simulink model "BrowarModel"  (R2024a)
settings: Solver=ode5  StartTime=0.0  StopTime=inf  FixedStep=0.1  RelTol=1e-3
undefined symbols (not defined in the file or in its folder): localhost, Matrikon, OI
libraries: opclib x24
(part 2 of 9)

== system BrowarModel/Kadz fermentacyjna/ET705 ==
  note: Przetwornik pomiarowy
  In : Inport
  F_gain : Gain  Gain=0
  F_offset : Constant  Value=0
  GUIMon : Gain
  Kompensacja : Constant  Value=Kompensacja
  Product : Product  RndMeth=Zero
  Saturation : Saturate  UpperLimit=100  LowerLimit=0
  Skalowanie (0-100%) : Gain  Gain=100/SrcZakres
  Sum{,1..3} (4 alike) : Sum  Inputs=|++
  Transfer Fcn : TransferFcn  Denominator=[0.3 1]
  Zaklocenia pomiarowe : Subsystem
  Zakres : Constant  Value=Zakres/100
  Out : Outport
  wires:
  Saturation/1 -> Product/1
  GUIMon/1 -> Out/1
  In/1 -> Skalowanie (0-100%)/1
  Sum2/1 -> Sum3/1
  Sum3/1 -> Transfer Fcn/1
  Sum1/1 -> Sum2/1, F_gain/1
  Zaklocenia pomiarowe/1(Out) -> Sum1/2
  Skalowanie (0-100%)/1 -> Sum1/1
  Sum/1 -> GUIMon/1
  Kompensacja/1 -> Sum/2
  Zakres/1 -> Product/2
  Product/1 -> Sum/1
  F_gain/1 -> Sum2/2
  F_offset/1 -> Sum3/2
  Transfer Fcn/1 -> Saturation/1

== system BrowarModel/Kadz fermentacyjna/FV705 ==
  note: Sterowanie
  GUIMon : Gain
  Lokalne : Constant
  Wybor : Switch  Threshold=0.5  SaturateOnIntegerOverflow=off  InputSameDT=off
  Out : Outport
  wires:
  GUIMon/1 -> Out/1
  Wybor/1 -> GUIMon/1
  [TrybSter] -> Wybor/2
  [FV705] -> Wybor/1
  Lokalne/1 -> Wybor/3

== system BrowarModel/Kadz fermentacyjna/FV705SP ==
  note: Sterowanie
  GUIMon : Gain
  Lokalne : Constant  Value=100
  Wybor : Switch  Threshold=0.5  SaturateOnIntegerOverflow=off  InputSameDT=off
  Out : Outport
  wires:
  Lokalne/1 -> Wybor/3
  [FV705SP] -> Wybor/1
  [TrybSter] -> Wybor/2
  Wybor/1 -> GUIMon/1
  GUIMon/1 -> Out/1

== system BrowarModel/Kadz fermentacyjna/FV706 ==
  note: Sterowanie
  GUIMon : Gain
  Lokalne : Constant
  Wybor : Switch  Threshold=0.5  SaturateOnIntegerOverflow=off  InputSameDT=off
  Out : Outport
  wires:
  GUIMon/1 -> Out/1
  Wybor/1 -> GUIMon/1
  [TrybSter] -> Wybor/2
  [FV706] -> Wybor/1
  Lokalne/1 -> Wybor/3

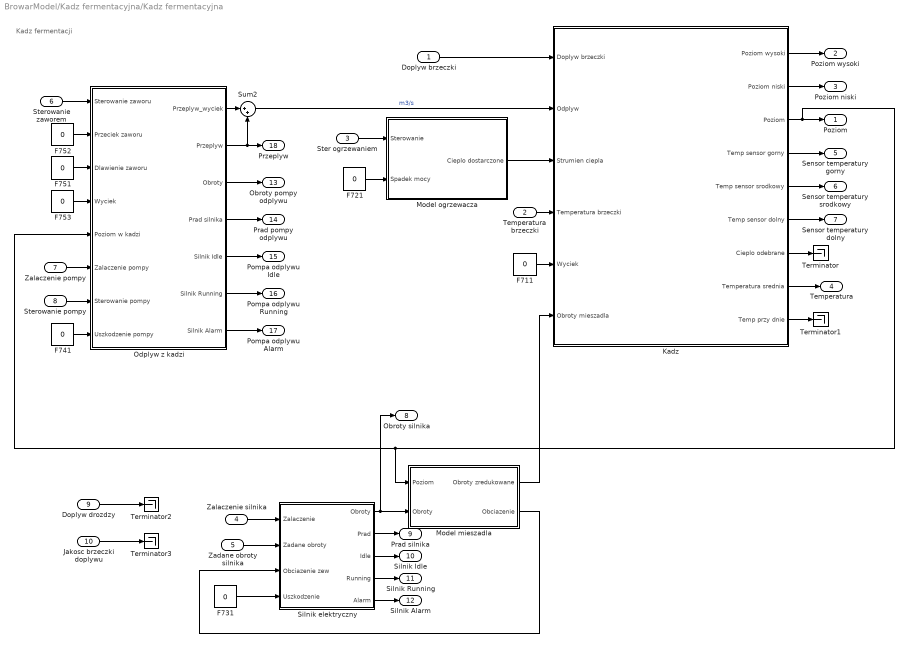
== system BrowarModel/Kadz fermentacyjna/Kadz fermentacyjna ==
  note: Kadz fermentacji
  Doplyw brzeczki : Inport
  Temperatura brzeczki : Inport  Port=2
  Ster ogrzewaniem : Inport  Port=3
  Zalaczenie silnika : Inport  Port=4
  "Zadane obroty silnika " : Inport  Port=5
  Sterowanie zaworem : Inport  Port=6
  Zalaczenie pompy : Inport  Port=7
  Sterowanie pompy : Inport  Port=8
  Doplyw drozdzy : Inport  Port=9
  Jakosc brzeczki doplywu : Inport  Port=10
  F{711,721,731,741,751..753} (7 alike) : Constant  Value=0
  Kadz : Subsystem
  Model mieszadla : Subsystem
  Model ogrzewacza : Subsystem
  Odplyw z kadzi : Subsystem
  Silnik elektryczny : Subsystem
  Sum2 : Sum  Inputs=|++
  Terminator{,1..3} (4 alike) : Terminator
  Poziom : Outport
  Poziom wysoki : Outport  Port=2
  Poziom niski : Outport  Port=3
  Temperatura : Outport  Port=4
  Sensor temperatury gorny : Outport  Port=5
  Sensor temperatury srodkowy : Outport  Port=6
  Sensor temperatury dolny : Outport  Port=7
  Obroty silnika : Outport  Port=8
  Prad silnika : Outport  Port=9
  Silnik Idle : Outport  Port=10
  Silnik Running : Outport  Port=11
  Silnik Alarm : Outport  Port=12
  Obroty pompy odplywu : Outport  Port=13
  Prad pompy odplywu : Outport  Port=14
  Pompa odplywu Idle : Outport  Port=15
  Pompa odplywu Running : Outport  Port=16
  Pompa odplywu Alarm : Outport  Port=17
  Przeplyw : Outport  Port=18
  wires:
  Model ogrzewacza/1(Cieplo dostarczone) -> Kadz/3(Strumien ciepla)
  Kadz/6(Temp sensor dolny) -> Sensor temperatury dolny/1
  Kadz/5(Temp sensor srodkowy) -> Sensor temperatury srodkowy/1
  Kadz/4(Temp sensor gorny) -> Sensor temperatury gorny/1
  Kadz/2(Poziom niski) -> Poziom niski/1
  Kadz/1(Poziom wysoki) -> Poziom wysoki/1
  Doplyw brzeczki/1 -> Kadz/1(Doplyw brzeczki)
  Temperatura brzeczki/1 -> Kadz/4(Temperatura brzeczki)
  Model mieszadla/1(Obroty zredukowane) -> Kadz/6(Obroty mieszadla)
  Kadz/3(Poziom) -> Poziom/1, Model mieszadla/1(Poziom), Odplyw z kadzi/5(Poziom w kadzi)
  Sum2/1 -> Kadz/2(Odplyw)  "m3/s"
  Kadz/8(Temperatura srednia) -> Temperatura/1
  F711/1 -> Kadz/5(Wyciek)
  Kadz/7(Cieplo odebrane) -> Terminator/1
  Silnik elektryczny/1(Obroty) -> Obroty silnika/1, Model mieszadla/2(Obroty)
  Ster ogrzewaniem/1 -> Model ogrzewacza/1(Sterowanie)
  F721/1 -> Model ogrzewacza/2(Spadek mocy)
  Kadz/9(Temp przy dnie) -> Terminator1/1
  Silnik elektryczny/3(Idle) -> Silnik Idle/1
  Silnik elektryczny/4(Running) -> Silnik Running/1
  Silnik elektryczny/5(Alarm) -> Silnik Alarm/1
  Silnik elektryczny/2(Prad) -> Prad silnika/1
  F731/1 -> Silnik elektryczny/4(Uszkodzenie)
  "Zadane obroty silnika "/1 -> Silnik elektryczny/2(Zadane obroty)
  Zalaczenie silnika/1 -> Silnik elektryczny/1(Zalaczenie)
  F752/1 -> Odplyw z kadzi/2(Przeciek zaworu)
  F751/1 -> Odplyw z kadzi/3(Dlawienie zaworu)
  F741/1 -> Odplyw z kadzi/8(Uszkodzenie pompy)
  Sterowanie zaworem/1 -> Odplyw z kadzi/1(Sterowanie zaworu)
  Zalaczenie pompy/1 -> Odplyw z kadzi/6(Zalaczenie pompy)
  Sterowanie pompy/1 -> Odplyw z kadzi/7(Sterowanie pompy)
  F753/1 -> Odplyw z kadzi/4(Wyciek)
  Odplyw z kadzi/4(Prad silnika) -> Prad pompy odplywu/1
  Odplyw z kadzi/5(Silnik Idle) -> Pompa odplywu Idle/1
  Odplyw z kadzi/6(Silnik Running) -> Pompa odplywu Running/1
  Odplyw z kadzi/7(Silnik Alarm) -> Pompa odplywu Alarm/1
  Odplyw z kadzi/3(Obroty) -> Obroty pompy odplywu/1
  Odplyw z kadzi/2(Przeplyw) -> Sum2/2, Przeplyw/1
  Odplyw z kadzi/1(Przeplyw_wyciek) -> Sum2/1
  Model mieszadla/2(Obciazenie) -> Silnik elektryczny/3(Obciazenie zew)
  Doplyw drozdzy/1 -> Terminator2/1
  Jakosc brzeczki doplywu/1 -> Terminator3/1

== system BrowarModel/Kadz fermentacyjna/LT701 ==
  note: Przetwornik pomiarowy
  In : Inport
  F_gain : Gain  Gain=0
  F_offset : Constant  Value=0
  GUIMon : Gain
  Kompensacja : Constant  Value=Kompensacja
  Product : Product  RndMeth=Zero
  Saturation : Saturate  UpperLimit=100  LowerLimit=0
  Skalowanie (0-100%) : Gain  Gain=100/SrcZakres
  Sum{,1..3} (4 alike) : Sum  Inputs=|++
  Transfer Fcn : TransferFcn  Denominator=[0.3 1]
  Zaklocenia pomiarowe : Subsystem
  Zakres : Constant  Value=Zakres/100
  Out : Outport
  wires:
  Saturation/1 -> Product/1
  GUIMon/1 -> Out/1
  In/1 -> Skalowanie (0-100%)/1
  Sum2/1 -> Sum3/1
  Sum3/1 -> Transfer Fcn/1
  Sum1/1 -> Sum2/1, F_gain/1
  Zaklocenia pomiarowe/1(Out) -> Sum1/2
  Skalowanie (0-100%)/1 -> Sum1/1
  Sum/1 -> GUIMon/1
  Kompensacja/1 -> Sum/2
  Zakres/1 -> Product/2
  Product/1 -> Sum/1
  F_gain/1 -> Sum2/2
  F_offset/1 -> Sum3/2
  Transfer Fcn/1 -> Saturation/1

== system BrowarModel/Kadz fermentacyjna/LT701H ==
  note: Przetwornik pomiarowy
  In : Inport
  FT : Constant  Value=0
  FT_value : Constant  Value=0
  GUIMon : Gain
  Switch : Switch  Threshold=0.5  SaturateOnIntegerOverflow=off  InputSameDT=off
  Out : Outport
  wires:
  In/1 -> Switch/3
  GUIMon/1 -> Out/1
  FT/1 -> Switch/2
  Switch/1 -> GUIMon/1
  FT_value/1 -> Switch/1

== system BrowarModel/Kadz fermentacyjna/LT701L ==
  note: Przetwornik pomiarowy
  In : Inport
  FT : Constant  Value=0
  FT_value : Constant  Value=0
  GUIMon : Gain
  Switch : Switch  Threshold=0.5  SaturateOnIntegerOverflow=off  InputSameDT=off
  Out : Outport
  wires:
  FT_value/1 -> Switch/1
  Switch/1 -> GUIMon/1
  FT/1 -> Switch/2
  GUIMon/1 -> Out/1
  In/1 -> Switch/3

== system BrowarModel/Kadz fermentacyjna/ST704 ==
  note: Przetwornik pomiarowy
  In : Inport
  F_gain : Gain  Gain=0
  F_offset : Constant  Value=0
  GUIMon : Gain
  Kompensacja : Constant  Value=Kompensacja
  Product : Product  RndMeth=Zero
  Saturation : Saturate  UpperLimit=100  LowerLimit=0
  Skalowanie (0-100%) : Gain  Gain=100/SrcZakres
  Sum{,1..3} (4 alike) : Sum  Inputs=|++
  Transfer Fcn : TransferFcn  Denominator=[0.3 1]
  Zaklocenia pomiarowe : Subsystem
  Zakres : Constant  Value=Zakres/100
  Out : Outport
  wires:
  Saturation/1 -> Product/1
  GUIMon/1 -> Out/1
  In/1 -> Skalowanie (0-100%)/1
  Sum2/1 -> Sum3/1
  Sum3/1 -> Transfer Fcn/1
  Sum1/1 -> Sum2/1, F_gain/1
  Zaklocenia pomiarowe/1(Out) -> Sum1/2
  Skalowanie (0-100%)/1 -> Sum1/1
  Sum/1 -> GUIMon/1
  Kompensacja/1 -> Sum/2
  Zakres/1 -> Product/2
  Product/1 -> Sum/1
  F_gain/1 -> Sum2/2
  F_offset/1 -> Sum3/2
  Transfer Fcn/1 -> Saturation/1

== system BrowarModel/Kadz fermentacyjna/ST705 ==
  note: Przetwornik pomiarowy
  In : Inport
  F_gain : Gain  Gain=0
  F_offset : Constant  Value=0
  GUIMon : Gain
  Kompensacja : Constant  Value=Kompensacja
  Product : Product  RndMeth=Zero
  Saturation : Saturate  UpperLimit=100  LowerLimit=0
  Skalowanie (0-100%) : Gain  Gain=100/SrcZakres
  Sum{,1..3} (4 alike) : Sum  Inputs=|++
  Transfer Fcn : TransferFcn  Denominator=[0.3 1]
  Zaklocenia pomiarowe : Subsystem
  Zakres : Constant  Value=Zakres/100
  Out : Outport
  wires:
  Transfer Fcn/1 -> Saturation/1
  F_offset/1 -> Sum3/2
  F_gain/1 -> Sum2/2
  Product/1 -> Sum/1
  Zakres/1 -> Product/2
  Kompensacja/1 -> Sum/2
  Sum/1 -> GUIMon/1
  Skalowanie (0-100%)/1 -> Sum1/1
  Zaklocenia pomiarowe/1(Out) -> Sum1/2
  Sum1/1 -> F_gain/1, Sum2/1
  Sum3/1 -> Transfer Fcn/1
  Sum2/1 -> Sum3/1
  In/1 -> Skalowanie (0-100%)/1
  GUIMon/1 -> Out/1
  Saturation/1 -> Product/1

== system BrowarModel/Kadz fermentacyjna/TT702H ==
  note: Przetwornik pomiarowy
  In : Inport
  F_gain : Gain  Gain=0
  F_offset : Constant  Value=0
  GUIMon : Gain
  Kompensacja : Constant  Value=Kompensacja
  Product : Product  RndMeth=Zero
  Saturation : Saturate  UpperLimit=100  LowerLimit=0
  Skalowanie (0-100%) : Gain  Gain=100/SrcZakres
  Sum{,1..3} (4 alike) : Sum  Inputs=|++
  Transfer Fcn : TransferFcn  Denominator=[0.3 1]
  Zaklocenia pomiarowe : Subsystem
  Zakres : Constant  Value=Zakres/100
  Out : Outport
  wires:
  Transfer Fcn/1 -> Saturation/1
  F_offset/1 -> Sum3/2
  F_gain/1 -> Sum2/2
  Product/1 -> Sum/1
  Zakres/1 -> Product/2
  Kompensacja/1 -> Sum/2
  Sum/1 -> GUIMon/1
  Skalowanie (0-100%)/1 -> Sum1/1
  Zaklocenia pomiarowe/1(Out) -> Sum1/2
  Sum1/1 -> F_gain/1, Sum2/1
  Sum3/1 -> Transfer Fcn/1
  Sum2/1 -> Sum3/1
  In/1 -> Skalowanie (0-100%)/1
  GUIMon/1 -> Out/1
  Saturation/1 -> Product/1

== system BrowarModel/Kadz fermentacyjna/TT702L ==
  note: Przetwornik pomiarowy
  In : Inport
  F_gain : Gain  Gain=0
  F_offset : Constant  Value=0
  GUIMon : Gain
  Kompensacja : Constant  Value=Kompensacja
  Product : Product  RndMeth=Zero
  Saturation : Saturate  UpperLimit=100  LowerLimit=0
  Skalowanie (0-100%) : Gain  Gain=100/SrcZakres
  Sum{,1..3} (4 alike) : Sum  Inputs=|++
  Transfer Fcn : TransferFcn  Denominator=[0.3 1]
  Zaklocenia pomiarowe : Subsystem
  Zakres : Constant  Value=Zakres/100
  Out : Outport
  wires:
  Transfer Fcn/1 -> Saturation/1
  F_offset/1 -> Sum3/2
  F_gain/1 -> Sum2/2
  Product/1 -> Sum/1
  Zakres/1 -> Product/2
  Kompensacja/1 -> Sum/2
  Sum/1 -> GUIMon/1
  Skalowanie (0-100%)/1 -> Sum1/1
  Zaklocenia pomiarowe/1(Out) -> Sum1/2
  Sum1/1 -> F_gain/1, Sum2/1
  Sum3/1 -> Transfer Fcn/1
  Sum2/1 -> Sum3/1
  In/1 -> Skalowanie (0-100%)/1
  GUIMon/1 -> Out/1
  Saturation/1 -> Product/1

== system BrowarModel/Kadz fermentacyjna/TT702M ==
  note: Przetwornik pomiarowy
  In : Inport
  F_gain : Gain  Gain=0
  F_offset : Constant  Value=0
  GUIMon : Gain
  Kompensacja : Constant  Value=Kompensacja
  Product : Product  RndMeth=Zero
  Saturation : Saturate  UpperLimit=100  LowerLimit=0
  Skalowanie (0-100%) : Gain  Gain=100/SrcZakres
  Sum{,1..3} (4 alike) : Sum  Inputs=|++
  Transfer Fcn : TransferFcn  Denominator=[0.3 1]
  Zaklocenia pomiarowe : Subsystem
  Zakres : Constant  Value=Zakres/100
  Out : Outport
  wires:
  Saturation/1 -> Product/1
  GUIMon/1 -> Out/1
  In/1 -> Skalowanie (0-100%)/1
  Sum2/1 -> Sum3/1
  Sum3/1 -> Transfer Fcn/1
  Sum1/1 -> Sum2/1, F_gain/1
  Zaklocenia pomiarowe/1(Out) -> Sum1/2
  Skalowanie (0-100%)/1 -> Sum1/1
  Sum/1 -> GUIMon/1
  Kompensacja/1 -> Sum/2
  Zakres/1 -> Product/2
  Product/1 -> Sum/1
  F_gain/1 -> Sum2/2
  F_offset/1 -> Sum3/2
  Transfer Fcn/1 -> Saturation/1

== system BrowarModel/Kadz fermentacyjna/TV702 ==
  note: Sterowanie
  GUIMon : Gain
  Lokalne : Constant  Value=0
  Wybor : Switch  Threshold=0.5  SaturateOnIntegerOverflow=off  InputSameDT=off
  Out : Outport
  wires:
  GUIMon/1 -> Out/1
  Wybor/1 -> GUIMon/1
  [TrybSter] -> Wybor/2
  [TV702] -> Wybor/1
  Lokalne/1 -> Wybor/3

== system BrowarModel/Kadz fermentacyjna/XV704 ==
  note: Sterowanie
  GUIMon : Gain
  Lokalne : Constant
  Wybor : Switch  Threshold=0.5  SaturateOnIntegerOverflow=off  InputSameDT=off
  Out : Outport
  wires:
  Lokalne/1 -> Wybor/3
  [XV704] -> Wybor/1
  [TrybSter] -> Wybor/2
  Wybor/1 -> GUIMon/1
  GUIMon/1 -> Out/1

== system BrowarModel/Kadz fermentacyjna/XV704SP ==
  note: Sterowanie
  GUIMon : Gain
  Lokalne : Constant  Value=100
  Wybor : Switch  Threshold=0.5  SaturateOnIntegerOverflow=off  InputSameDT=off
  Out : Outport
  wires:
  GUIMon/1 -> Out/1
  Wybor/1 -> GUIMon/1
  [TrybSter] -> Wybor/2
  [XV704SP] -> Wybor/1
  Lokalne/1 -> Wybor/3

== system BrowarModel/Kadz filtracji/ET302 ==
  note: Przetwornik pomiarowy
  In : Inport
  F_gain : Gain  Gain=0
  F_offset : Constant  Value=0
  GUIMon : Gain
  Kompensacja : Constant  Value=Kompensacja
  Product : Product  RndMeth=Zero
  Saturation : Saturate  UpperLimit=100  LowerLimit=0
  Skalowanie (0-100%) : Gain  Gain=100/SrcZakres
  Sum{,1..3} (4 alike) : Sum  Inputs=|++
  Transfer Fcn : TransferFcn  Denominator=[0.3 1]
  Zaklocenia pomiarowe : Subsystem
  Zakres : Constant  Value=Zakres/100
  Out : Outport
  wires:
  Transfer Fcn/1 -> Saturation/1
  F_offset/1 -> Sum3/2
  F_gain/1 -> Sum2/2
  Product/1 -> Sum/1
  Zakres/1 -> Product/2
  Kompensacja/1 -> Sum/2
  Sum/1 -> GUIMon/1
  Skalowanie (0-100%)/1 -> Sum1/1
  Zaklocenia pomiarowe/1(Out) -> Sum1/2
  Sum1/1 -> F_gain/1, Sum2/1
  Sum3/1 -> Transfer Fcn/1
  Sum2/1 -> Sum3/1
  In/1 -> Skalowanie (0-100%)/1
  GUIMon/1 -> Out/1
  Saturation/1 -> Product/1

== system BrowarModel/Kadz filtracji/ET304 ==
  note: Przetwornik pomiarowy
  In : Inport
  F_gain : Gain  Gain=0
  F_offset : Constant  Value=0
  GUIMon : Gain
  Kompensacja : Constant  Value=Kompensacja
  Product : Product  RndMeth=Zero
  Saturation : Saturate  UpperLimit=100  LowerLimit=0
  Skalowanie (0-100%) : Gain  Gain=100/SrcZakres
  Sum{,1..3} (4 alike) : Sum  Inputs=|++
  Transfer Fcn : TransferFcn  Denominator=[0.3 1]
  Zaklocenia pomiarowe : Subsystem
  Zakres : Constant  Value=Zakres/100
  Out : Outport
  wires:
  Saturation/1 -> Product/1
  GUIMon/1 -> Out/1
  In/1 -> Skalowanie (0-100%)/1
  Sum2/1 -> Sum3/1
  Sum3/1 -> Transfer Fcn/1
  Sum1/1 -> Sum2/1, F_gain/1
  Zaklocenia pomiarowe/1(Out) -> Sum1/2
  Skalowanie (0-100%)/1 -> Sum1/1
  Sum/1 -> GUIMon/1
  Kompensacja/1 -> Sum/2
  Zakres/1 -> Product/2
  Product/1 -> Sum/1
  F_gain/1 -> Sum2/2
  F_offset/1 -> Sum3/2
  Transfer Fcn/1 -> Saturation/1

== system BrowarModel/Kadz filtracji/ET307 ==
  note: Przetwornik pomiarowy
  In : Inport
  F_gain : Gain  Gain=0
  F_offset : Constant  Value=0
  GUIMon : Gain
  Kompensacja : Constant  Value=Kompensacja
  Product : Product  RndMeth=Zero
  Saturation : Saturate  UpperLimit=100  LowerLimit=0
  Skalowanie (0-100%) : Gain  Gain=100/SrcZakres
  Sum{,1..3} (4 alike) : Sum  Inputs=|++
  Transfer Fcn : TransferFcn  Denominator=[0.3 1]
  Zaklocenia pomiarowe : Subsystem
  Zakres : Constant  Value=Zakres/100
  Out : Outport
  wires:
  Saturation/1 -> Product/1
  GUIMon/1 -> Out/1
  In/1 -> Skalowanie (0-100%)/1
  Sum2/1 -> Sum3/1
  Sum3/1 -> Transfer Fcn/1
  Sum1/1 -> Sum2/1, F_gain/1
  Zaklocenia pomiarowe/1(Out) -> Sum1/2
  Skalowanie (0-100%)/1 -> Sum1/1
  Sum/1 -> GUIMon/1
  Kompensacja/1 -> Sum/2
  Zakres/1 -> Product/2
  Product/1 -> Sum/1
  F_gain/1 -> Sum2/2
  F_offset/1 -> Sum3/2
  Transfer Fcn/1 -> Saturation/1

== system BrowarModel/Kadz filtracji/FV301 ==
  note: Sterowanie
  GUIMon : Gain
  Lokalne : Constant
  Wybor : Switch  Threshold=0.5  SaturateOnIntegerOverflow=off  InputSameDT=off
  Out : Outport
  wires:
  Lokalne/1 -> Wybor/3
  [FV301] -> Wybor/1
  [TrybSter] -> Wybor/2
  Wybor/1 -> GUIMon/1
  GUIMon/1 -> Out/1

== system BrowarModel/Kadz filtracji/FV302 ==
  note: Sterowanie
  GUIMon : Gain
  Lokalne : Constant  Value=0
  Wybor : Switch  Threshold=0.5  SaturateOnIntegerOverflow=off  InputSameDT=off
  Out : Outport
  wires:
  GUIMon/1 -> Out/1
  Wybor/1 -> GUIMon/1
  [TrybSter] -> Wybor/2
  [FV302] -> Wybor/1
  Lokalne/1 -> Wybor/3

== system BrowarModel/Kadz filtracji/FV302SP ==
  note: Sterowanie
  GUIMon : Gain
  Lokalne : Constant  Value=100
  Wybor : Switch  Threshold=0.5  SaturateOnIntegerOverflow=off  InputSameDT=off
  Out : Outport
  wires:
  Lokalne/1 -> Wybor/3
  [FV302SP] -> Wybor/1
  [TrybSter] -> Wybor/2
  Wybor/1 -> GUIMon/1
  GUIMon/1 -> Out/1

== system BrowarModel/Kadz filtracji/FV303 ==
  note: Sterowanie
  GUIMon : Gain
  Lokalne : Constant  Value=0
  Wybor : Switch  Threshold=0.5  SaturateOnIntegerOverflow=off  InputSameDT=off
  Out : Outport
  wires:
  GUIMon/1 -> Out/1
  Wybor/1 -> GUIMon/1
  [TrybSter] -> Wybor/2
  [FV303] -> Wybor/1
  Lokalne/1 -> Wybor/3

== system BrowarModel/Kadz filtracji/FV304 ==
  note: Sterowanie
  GUIMon : Gain
  Lokalne : Constant
  Wybor : Switch  Threshold=0.5  SaturateOnIntegerOverflow=off  InputSameDT=off
  Out : Outport
  wires:
  Lokalne/1 -> Wybor/3
  [FV304] -> Wybor/1
  [TrybSter] -> Wybor/2
  Wybor/1 -> GUIMon/1
  GUIMon/1 -> Out/1

== system BrowarModel/Kadz filtracji/FV304SP ==
  note: Sterowanie
  GUIMon : Gain
  Lokalne : Constant  Value=100
  Wybor : Switch  Threshold=0.5  SaturateOnIntegerOverflow=off  InputSameDT=off
  Out : Outport
  wires:
  GUIMon/1 -> Out/1
  Wybor/1 -> GUIMon/1
  [TrybSter] -> Wybor/2
  [FV304SP] -> Wybor/1
  Lokalne/1 -> Wybor/3

== system BrowarModel/Kadz filtracji/FV305 ==
  note: Sterowanie
  GUIMon : Gain
  Lokalne : Constant
  Wybor : Switch  Threshold=0.5  SaturateOnIntegerOverflow=off  InputSameDT=off
  Out : Outport
  wires:
  GUIMon/1 -> Out/1
  Wybor/1 -> GUIMon/1
  [TrybSter] -> Wybor/2
  [FV305] -> Wybor/1
  Lokalne/1 -> Wybor/3

== system BrowarModel/Kadz filtracji/FV306 ==
  note: Sterowanie
  GUIMon : Gain
  Lokalne : Constant  Value=0
  Wybor : Switch  Threshold=0.5  SaturateOnIntegerOverflow=off  InputSameDT=off
  Out : Outport
  wires:
  Lokalne/1 -> Wybor/3
  [FV306] -> Wybor/1
  [TrybSter] -> Wybor/2
  Wybor/1 -> GUIMon/1
  GUIMon/1 -> Out/1

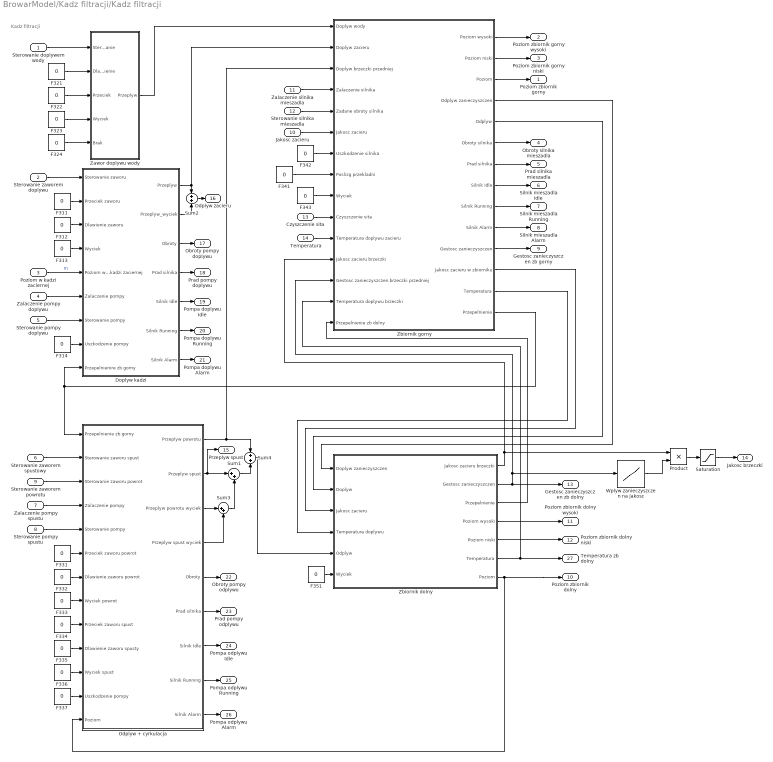
== system BrowarModel/Kadz filtracji/Kadz filtracji ==
  note: Kadz filtracji
  Sterowanie doplywem wody : Inport
  Sterowanie zaworem doplywu : Inport  Port=2
  Poziom w kadzi zaciernej : Inport  Port=3
  Zalaczenie pompy doplywu : Inport  Port=4
  Sterowanie pompy doplywu : Inport  Port=5
  Sterowanie zaworem spustowy : Inport  Port=6
  Zalaczenie pompy spustu : Inport  Port=7
  Sterowanie pompy spustu : Inport  Port=8
  Sterowanie zaworem powrotu : Inport  Port=9
  Jakosc zacieru : Inport  Port=10
  Zalaczenie silnika mieszadla : Inport  Port=11
  Sterowanie silnika mieszadla : Inport  Port=12
  Czyszczenie sita : Inport  Port=13
  Temperatura : Inport  Port=14
  Doplyw kadzi : Subsystem
  F{311..314,321..324,331..337,341..343,351} (19 alike) : Constant  Value=0
  Odplyw + cyrkulacja : Subsystem
  Product : Product  RndMeth=Zero
  Saturation : Saturate  UpperLimit=inf  LowerLimit=0
  Sum1 : Sum  Inputs=|++
  Sum2 : Sum
  Sum3 : Sum  Inputs=|++
  Sum4 : Sum
  Wplyw zanieczyszczen na jakosc : Lookup  InputValues=[0 0.05 0.1 0.2 0.5 1]  Table=[1 1 0.95 0.3 0.1 0.01]  SaturateOnIntegerOverflow=off
  Zawor doplywu wody : Subsystem  mask{Fmax=0.2}
      mask prompts: Fmax "Przeplyw maksymalny [m3/s]"
  Zbiornik dolny : Subsystem
  Zbiornik gorny : Subsystem
  Poziom zbiornik gorny : Outport
  Poziom zbiornik gorny wysoki : Outport  Port=2
  Poziom zbiornik gorny niski : Outport  Port=3
  Obroty silnika mieszadla : Outport  Port=4
  Prad silnika mieszadla : Outport  Port=5
  Silnik mieszadla Idle : Outport  Port=6
  Silnik mieszadla Running : Outport  Port=7
  Silnik mieszadla Alarm : Outport  Port=8
  Gestosc zanieczyszczen zb gorny : Outport  Port=9
  Poziom zbiornik dolny : Outport  Port=10
  Poziom zbiornik dolny wysoki : Outport  Port=11
  Poziom zbiornik dolny niski : Outport  Port=12
  Gestosc zanieczyszczen zb dolny : Outport  Port=13
  Jakosc brzeczki : Outport  Port=14
  Przeplyw spust : Outport  Port=15
  Odplyw zacieru : Outport  Port=16
  Obroty pompy doplywu : Outport  Port=17
  Prad pompy doplywu : Outport  Port=18
  Pompa doplywu Idle : Outport  Port=19
  Pompa doplywu Running : Outport  Port=20
  Pompa doplywu Alarm : Outport  Port=21
  Obroty pompy odplywu : Outport  Port=22
  Prad pompy odplywu : Outport  Port=23
  Pompa odplywu Idle : Outport  Port=24
  Pompa odplywu Running : Outport  Port=25
  Pompa odplywu Alarm : Outport  Port=26
  Temperatura zb dolny : Outport  Port=27
  wires:
  Zawor doplywu wody/1(Przeplyw) -> Zbiornik gorny/1(Doplyw wody)
  Zbiornik gorny/1(Poziom wysoki) -> Poziom zbiornik gorny wysoki/1
  Zbiornik gorny/2(Poziom niski) -> Poziom zbiornik gorny niski/1
  Zbiornik dolny/4(Poziom wysoki) -> Poziom zbiornik dolny wysoki/1
  Zbiornik dolny/5(Poziom niski) -> Poziom zbiornik dolny niski/1
  Zbiornik dolny/7(Poziom) -> Odplyw + cyrkulacja/13(Poziom), Poziom zbiornik dolny/1
  Zbiornik gorny/4(Odplyw zanieczyszczen) -> Zbiornik dolny/1(Doplyw zanieczyszczen)
  Zbiornik dolny/2(Gestosc zanieczyszczen) -> Gestosc zanieczyszczen zb dolny/1, Zbiornik gorny/13(Gestosc zanieczyszczen brzeczki przedniej), Wplyw zanieczyszczen na jakosc/1
  Zbiornik gorny/3(Poziom) -> Poziom zbiornik gorny/1
  Zbiornik gorny/5(Odplyw) -> Zbiornik dolny/2(Doplyw)
  F311/1 -> Doplyw kadzi/2(Przeciek zaworu)
  F312/1 -> Doplyw kadzi/3(Dlawienie zaworu)
  F314/1 -> Doplyw kadzi/8(Uszkodzenie pompy)
  Sterowanie zaworem doplywu/1 -> Doplyw kadzi/1(Sterowanie zaworu)
  Poziom w kadzi zaciernej/1 -> Doplyw kadzi/5(Poziom w kadzi zaciernej)  "m"
  Zalaczenie pompy doplywu/1 -> Doplyw kadzi/6(Zalaczenie pompy)
  Sterowanie pompy doplywu/1 -> Doplyw kadzi/7(Sterowanie pompy)
  Doplyw kadzi/1(Przeplyw) -> Sum2/1, Zbiornik gorny/2(Doplyw zacieru)
  Sterowanie zaworem spustowy/1 -> Odplyw + cyrkulacja/2(Sterowanie zaworu spust)
  Zalaczenie pompy spustu/1 -> Odplyw + cyrkulacja/4(Zalaczenie pompy)
  Sterowanie pompy spustu/1 -> Odplyw + cyrkulacja/5(Sterowanie pompy)
  Sterowanie zaworem powrotu/1 -> Odplyw + cyrkulacja/3(Sterowanie zaworu powrot)
  Product/1 -> Saturation/1
  Odplyw + cyrkulacja/2(Przeplyw spust) -> Sum1/1, Przeplyw spust/1
  F342/1 -> Zbiornik gorny/7(Uszkodzenie silnika)
  F341/1 -> Zbiornik gorny/8(Poslizg przekladni)
  F343/1 -> Zbiornik gorny/9(Wyciek)
  F351/1 -> Zbiornik dolny/6(Wyciek)
  Doplyw kadzi/2(Przeplyw_wyciek) -> Sum2/2
  Sum2/1 -> Odplyw zacieru/1
  Odplyw + cyrkulacja/1(Przeplyw powrotu) -> Sum4/1, Zbiornik gorny/3(Doplyw brzeczki przedniej)
  Odplyw + cyrkulacja/3(Przeplyw powrotu wyciek) -> Sum3/1
  Odplyw + cyrkulacja/4(Przeplyw spust wyciek) -> Sum3/2
  Sum4/1 -> Zbiornik dolny/5(Odplyw)
  Sum3/1 -> Sum1/2
  Sum1/1 -> Sum4/2
  F331/1 -> Odplyw + cyrkulacja/6(Przeciek zaworu powrot)
  F332/1 -> Odplyw + cyrkulacja/7(Dlawienie zaworu powrot)
  F333/1 -> Odplyw + cyrkulacja/8(Wyciek powrot)
  F334/1 -> Odplyw + cyrkulacja/9(Przeciek zaworu spust)
  F335/1 -> Odplyw + cyrkulacja/10(Dlawienie zaworu spusty)
  F336/1 -> Odplyw + cyrkulacja/11(Wyciek spust)
  F337/1 -> Odplyw + cyrkulacja/12(Uszkodzenie pompy)
  Zbiornik dolny/1(Jakosc zacieru brzeczki) -> Zbiornik gorny/12(Jakosc zacieru brzeczki), Product/1
  Zbiornik gorny/12(Jakosc zacieru w zbiorniku) -> Zbiornik dolny/3(Jakosc zacieru)
  Jakosc zacieru/1 -> Zbiornik gorny/6(Jakosc zacieru)
  Zalaczenie silnika mieszadla/1 -> Zbiornik gorny/4(Zalaczenie silnika)
  Sterowanie silnika mieszadla/1 -> Zbiornik gorny/5("Zadane obroty silnika ")
  Zbiornik gorny/6(Obroty silnika) -> Obroty silnika mieszadla/1
  Zbiornik gorny/7(Prad silnika) -> Prad silnika mieszadla/1
  Zbiornik gorny/11(Gestosc zanieczyszczen) -> Gestosc zanieczyszczen zb gorny/1
  Wplyw zanieczyszczen na jakosc/1 -> Product/2
  Saturation/1 -> Jakosc brzeczki/1
  F313/1 -> Doplyw kadzi/4(Wyciek)
  Zbiornik gorny/8(Silnik Idle) -> Silnik mieszadla Idle/1
  Zbiornik gorny/9(Silnik Running) -> Silnik mieszadla Running/1
  Zbiornik gorny/10(Silnik Alarm) -> Silnik mieszadla Alarm/1
  Sterowanie doplywem wody/1 -> Zawor doplywu wody/1(Sterowanie)
  F321/1 -> Zawor doplywu wody/2(Dlawienie)
  F322/1 -> Zawor doplywu wody/3(Przeciek)
  F323/1 -> Zawor doplywu wody/4(Wyciek)
  F324/1 -> Zawor doplywu wody/5(Brak)
  Czyszczenie sita/1 -> Zbiornik gorny/10(Czyszczenie sita)
  Doplyw kadzi/4(Prad silnika) -> Prad pompy doplywu/1
  Doplyw kadzi/5(Silnik Idle) -> Pompa doplywu Idle/1
  Doplyw kadzi/6(Silnik Running) -> Pompa doplywu Running/1
  Doplyw kadzi/7(Silnik Alarm) -> Pompa doplywu Alarm/1
  Doplyw kadzi/3(Obroty) -> Obroty pompy doplywu/1
  Odplyw + cyrkulacja/5(Obroty) -> Obroty pompy odplywu/1
  Odplyw + cyrkulacja/6(Prad silnika) -> Prad pompy odplywu/1
  Odplyw + cyrkulacja/7(Silnik Idle) -> Pompa odplywu Idle/1
  Odplyw + cyrkulacja/8(Silnik Running) -> Pompa odplywu Running/1
  Odplyw + cyrkulacja/9(Silnik Alarm) -> Pompa odplywu Alarm/1
  Zbiornik dolny/6(Temperatura) -> Temperatura zb dolny/1, Zbiornik gorny/14(Temperatura doplywu brzeczki)
  Temperatura/1 -> Zbiornik gorny/11(Temperatura doplywu zacieru)
  Zbiornik gorny/13(Temperatura) -> Zbiornik dolny/4(Temperatura doplywu)
  Zbiornik gorny/14(Przepelnienie) -> Doplyw kadzi/9(Przepelnienire zb gorny), Odplyw + cyrkulacja/1(Przepelnienie zb gorny)
  Zbiornik dolny/3(Przepelnienie) -> Zbiornik gorny/15(Przepelnienie zb dolny)

== system BrowarModel/Kadz filtracji/LT308 ==
  note: Przetwornik pomiarowy
  In : Inport
  F_gain : Gain  Gain=0
  F_offset : Constant  Value=0
  GUIMon : Gain
  Kompensacja : Constant  Value=Kompensacja
  Product : Product  RndMeth=Zero
  Saturation : Saturate  UpperLimit=100  LowerLimit=0
  Skalowanie (0-100%) : Gain  Gain=100/SrcZakres
  Sum{,1..3} (4 alike) : Sum  Inputs=|++
  Transfer Fcn : TransferFcn  Denominator=[0.3 1]
  Zaklocenia pomiarowe : Subsystem
  Zakres : Constant  Value=Zakres/100
  Out : Outport
  wires:
  Saturation/1 -> Product/1
  GUIMon/1 -> Out/1
  In/1 -> Skalowanie (0-100%)/1
  Sum2/1 -> Sum3/1
  Sum3/1 -> Transfer Fcn/1
  Sum1/1 -> Sum2/1, F_gain/1
  Zaklocenia pomiarowe/1(Out) -> Sum1/2
  Skalowanie (0-100%)/1 -> Sum1/1
  Sum/1 -> GUIMon/1
  Kompensacja/1 -> Sum/2
  Zakres/1 -> Product/2
  Product/1 -> Sum/1
  F_gain/1 -> Sum2/2
  F_offset/1 -> Sum3/2
  Transfer Fcn/1 -> Saturation/1

== system BrowarModel/Kadz filtracji/LT308H ==
  note: Przetwornik pomiarowy
  In : Inport
  FT : Constant  Value=0
  FT_value : Constant  Value=0
  GUIMon : Gain
  Switch : Switch  Threshold=0.5  SaturateOnIntegerOverflow=off  InputSameDT=off
  Out : Outport
  wires:
  In/1 -> Switch/3
  GUIMon/1 -> Out/1
  FT/1 -> Switch/2
  Switch/1 -> GUIMon/1
  FT_value/1 -> Switch/1

== system BrowarModel/Kadz filtracji/LT308L ==
  note: Przetwornik pomiarowy
  In : Inport
  FT : Constant  Value=0
  FT_value : Constant  Value=0
  GUIMon : Gain
  Switch : Switch  Threshold=0.5  SaturateOnIntegerOverflow=off  InputSameDT=off
  Out : Outport
  wires:
  FT_value/1 -> Switch/1
  Switch/1 -> GUIMon/1
  FT/1 -> Switch/2
  GUIMon/1 -> Out/1
  In/1 -> Switch/3

== system BrowarModel/Kadz filtracji/LT309 ==
  note: Przetwornik pomiarowy
  In : Inport
  F_gain : Gain  Gain=0
  F_offset : Constant  Value=0
  GUIMon : Gain
  Kompensacja : Constant  Value=Kompensacja
  Product : Product  RndMeth=Zero
  Saturation : Saturate  UpperLimit=100  LowerLimit=0
  Skalowanie (0-100%) : Gain  Gain=100/SrcZakres
  Sum{,1..3} (4 alike) : Sum  Inputs=|++
  Transfer Fcn : TransferFcn  Denominator=[0.3 1]
  Zaklocenia pomiarowe : Subsystem
  Zakres : Constant  Value=Zakres/100
  Out : Outport
  wires:
  Transfer Fcn/1 -> Saturation/1
  F_offset/1 -> Sum3/2
  F_gain/1 -> Sum2/2
  Product/1 -> Sum/1
  Zakres/1 -> Product/2
  Kompensacja/1 -> Sum/2
  Sum/1 -> GUIMon/1
  Skalowanie (0-100%)/1 -> Sum1/1
  Zaklocenia pomiarowe/1(Out) -> Sum1/2
  Sum1/1 -> F_gain/1, Sum2/1
  Sum3/1 -> Transfer Fcn/1
  Sum2/1 -> Sum3/1
  In/1 -> Skalowanie (0-100%)/1
  GUIMon/1 -> Out/1
  Saturation/1 -> Product/1

== system BrowarModel/Kadz filtracji/LT309H ==
  note: Przetwornik pomiarowy
  In : Inport
  FT : Constant  Value=0
  FT_value : Constant  Value=0
  GUIMon : Gain
  Switch : Switch  Threshold=0.5  SaturateOnIntegerOverflow=off  InputSameDT=off
  Out : Outport
  wires:
  In/1 -> Switch/3
  GUIMon/1 -> Out/1
  FT/1 -> Switch/2
  Switch/1 -> GUIMon/1
  FT_value/1 -> Switch/1

== system BrowarModel/Kadz filtracji/LT309L ==
  note: Przetwornik pomiarowy
  In : Inport
  FT : Constant  Value=0
  FT_value : Constant  Value=0
  GUIMon : Gain
  Switch : Switch  Threshold=0.5  SaturateOnIntegerOverflow=off  InputSameDT=off
  Out : Outport
  wires:
  FT_value/1 -> Switch/1
  Switch/1 -> GUIMon/1
  FT/1 -> Switch/2
  GUIMon/1 -> Out/1
  In/1 -> Switch/3

== system BrowarModel/Kadz filtracji/QT310 ==
  note: Przetwornik pomiarowy
  In : Inport
  F_gain : Gain  Gain=0
  F_offset : Constant  Value=0
  GUIMon : Gain
  Kompensacja : Constant  Value=Kompensacja
  Product : Product  RndMeth=Zero
  Saturation : Saturate  UpperLimit=100  LowerLimit=0
  Skalowanie (0-100%) : Gain  Gain=100/SrcZakres
  Sum{,1..3} (4 alike) : Sum  Inputs=|++
  Transfer Fcn : TransferFcn  Denominator=[0.3 1]
  Zaklocenia pomiarowe : Subsystem
  Zakres : Constant  Value=Zakres/100
  Out : Outport
  wires:
  Transfer Fcn/1 -> Saturation/1
  F_offset/1 -> Sum3/2
  F_gain/1 -> Sum2/2
  Product/1 -> Sum/1
  Zakres/1 -> Product/2
  Kompensacja/1 -> Sum/2
  Sum/1 -> GUIMon/1
  Skalowanie (0-100%)/1 -> Sum1/1
  Zaklocenia pomiarowe/1(Out) -> Sum1/2
  Sum1/1 -> F_gain/1, Sum2/1
  Sum3/1 -> Transfer Fcn/1
  Sum2/1 -> Sum3/1
  In/1 -> Skalowanie (0-100%)/1
  GUIMon/1 -> Out/1
  Saturation/1 -> Product/1

== system BrowarModel/Kadz filtracji/QT311 ==
  note: Przetwornik pomiarowy
  In : Inport
  F_gain : Gain  Gain=0
  F_offset : Constant  Value=0
  GUIMon : Gain
  Kompensacja : Constant  Value=Kompensacja
  Product : Product  RndMeth=Zero
  Saturation : Saturate  UpperLimit=100  LowerLimit=0
  Skalowanie (0-100%) : Gain  Gain=100/SrcZakres
  Sum{,1..3} (4 alike) : Sum  Inputs=|++
  Transfer Fcn : TransferFcn  Denominator=[0.3 1]
  Zaklocenia pomiarowe : Subsystem
  Zakres : Constant  Value=Zakres/100
  Out : Outport
  wires:
  Saturation/1 -> Product/1
  GUIMon/1 -> Out/1
  In/1 -> Skalowanie (0-100%)/1
  Sum2/1 -> Sum3/1
  Sum3/1 -> Transfer Fcn/1
  Sum1/1 -> Sum2/1, F_gain/1
  Zaklocenia pomiarowe/1(Out) -> Sum1/2
  Skalowanie (0-100%)/1 -> Sum1/1
  Sum/1 -> GUIMon/1
  Kompensacja/1 -> Sum/2
  Zakres/1 -> Product/2
  Product/1 -> Sum/1
  F_gain/1 -> Sum2/2
  F_offset/1 -> Sum3/2
  Transfer Fcn/1 -> Saturation/1

== system BrowarModel/Kadz filtracji/QT312 ==
  note: Przetwornik pomiarowy
  In : Inport
  F_gain : Gain  Gain=0
  F_offset : Constant  Value=0
  GUIMon : Gain
  Kompensacja : Constant  Value=Kompensacja
  Product : Product  RndMeth=Zero
  Saturation : Saturate  UpperLimit=100  LowerLimit=0
  Skalowanie (0-100%) : Gain  Gain=100/SrcZakres
  Sum{,1..3} (4 alike) : Sum  Inputs=|++
  Transfer Fcn : TransferFcn  Denominator=[0.3 1]
  Zaklocenia pomiarowe : Subsystem
  Zakres : Constant  Value=Zakres/100
  Out : Outport
  wires:
  Transfer Fcn/1 -> Saturation/1
  F_offset/1 -> Sum3/2
  F_gain/1 -> Sum2/2
  Product/1 -> Sum/1
  Zakres/1 -> Product/2
  Kompensacja/1 -> Sum/2
  Sum/1 -> GUIMon/1
  Skalowanie (0-100%)/1 -> Sum1/1
  Zaklocenia pomiarowe/1(Out) -> Sum1/2
  Sum1/1 -> F_gain/1, Sum2/1
  Sum3/1 -> Transfer Fcn/1
  Sum2/1 -> Sum3/1
  In/1 -> Skalowanie (0-100%)/1
  GUIMon/1 -> Out/1
  Saturation/1 -> Product/1

== system BrowarModel/Kadz filtracji/ST302 ==
  note: Przetwornik pomiarowy
  In : Inport
  F_gain : Gain  Gain=0
  F_offset : Constant  Value=0
  GUIMon : Gain
  Kompensacja : Constant  Value=Kompensacja
  Product : Product  RndMeth=Zero
  Saturation : Saturate  UpperLimit=100  LowerLimit=0
  Skalowanie (0-100%) : Gain  Gain=100/SrcZakres
  Sum{,1..3} (4 alike) : Sum  Inputs=|++
  Transfer Fcn : TransferFcn  Denominator=[0.3 1]
  Zaklocenia pomiarowe : Subsystem
  Zakres : Constant  Value=Zakres/100
  Out : Outport
  wires:
  Saturation/1 -> Product/1
  GUIMon/1 -> Out/1
  In/1 -> Skalowanie (0-100%)/1
  Sum2/1 -> Sum3/1
  Sum3/1 -> Transfer Fcn/1
  Sum1/1 -> Sum2/1, F_gain/1
  Zaklocenia pomiarowe/1(Out) -> Sum1/2
  Skalowanie (0-100%)/1 -> Sum1/1
  Sum/1 -> GUIMon/1
  Kompensacja/1 -> Sum/2
  Zakres/1 -> Product/2
  Product/1 -> Sum/1
  F_gain/1 -> Sum2/2
  F_offset/1 -> Sum3/2
  Transfer Fcn/1 -> Saturation/1

== system BrowarModel/Kadz filtracji/ST304 ==
  note: Przetwornik pomiarowy
  In : Inport
  F_gain : Gain  Gain=0
  F_offset : Constant  Value=0
  GUIMon : Gain
  Kompensacja : Constant  Value=Kompensacja
  Product : Product  RndMeth=Zero
  Saturation : Saturate  UpperLimit=100  LowerLimit=0
  Skalowanie (0-100%) : Gain  Gain=100/SrcZakres
  Sum{,1..3} (4 alike) : Sum  Inputs=|++
  Transfer Fcn : TransferFcn  Denominator=[0.3 1]
  Zaklocenia pomiarowe : Subsystem
  Zakres : Constant  Value=Zakres/100
  Out : Outport
  wires:
  Transfer Fcn/1 -> Saturation/1
  F_offset/1 -> Sum3/2
  F_gain/1 -> Sum2/2
  Product/1 -> Sum/1
  Zakres/1 -> Product/2
  Kompensacja/1 -> Sum/2
  Sum/1 -> GUIMon/1
  Skalowanie (0-100%)/1 -> Sum1/1
  Zaklocenia pomiarowe/1(Out) -> Sum1/2
  Sum1/1 -> F_gain/1, Sum2/1
  Sum3/1 -> Transfer Fcn/1
  Sum2/1 -> Sum3/1
  In/1 -> Skalowanie (0-100%)/1
  GUIMon/1 -> Out/1
  Saturation/1 -> Product/1

== system BrowarModel/Kadz filtracji/ST307 ==
  note: Przetwornik pomiarowy
  In : Inport
  F_gain : Gain  Gain=0
  F_offset : Constant  Value=0
  GUIMon : Gain
  Kompensacja : Constant  Value=Kompensacja
  Product : Product  RndMeth=Zero
  Saturation : Saturate  UpperLimit=100  LowerLimit=0
  Skalowanie (0-100%) : Gain  Gain=100/SrcZakres
  Sum{,1..3} (4 alike) : Sum  Inputs=|++
  Transfer Fcn : TransferFcn  Denominator=[0.3 1]
  Zaklocenia pomiarowe : Subsystem
  Zakres : Constant  Value=Zakres/100
  Out : Outport
  wires:
  Transfer Fcn/1 -> Saturation/1
  F_offset/1 -> Sum3/2
  F_gain/1 -> Sum2/2
  Product/1 -> Sum/1
  Zakres/1 -> Product/2
  Kompensacja/1 -> Sum/2
  Sum/1 -> GUIMon/1
  Skalowanie (0-100%)/1 -> Sum1/1
  Zaklocenia pomiarowe/1(Out) -> Sum1/2
  Sum1/1 -> F_gain/1, Sum2/1
  Sum3/1 -> Transfer Fcn/1
  Sum2/1 -> Sum3/1
  In/1 -> Skalowanie (0-100%)/1
  GUIMon/1 -> Out/1
  Saturation/1 -> Product/1

== system BrowarModel/Kadz filtracji/XV307 ==
  note: Sterowanie
  GUIMon : Gain
  Lokalne : Constant  Value=0
  Wybor : Switch  Threshold=0.5  SaturateOnIntegerOverflow=off  InputSameDT=off
  Out : Outport
  wires:
  GUIMon/1 -> Out/1
  Wybor/1 -> GUIMon/1
  [TrybSter] -> Wybor/2
  [XV307] -> Wybor/1
  Lokalne/1 -> Wybor/3

== system BrowarModel/Kadz filtracji/XV307SP ==
  note: Sterowanie
  GUIMon : Gain
  Lokalne : Constant  Value=100
  Wybor : Switch  Threshold=0.5  SaturateOnIntegerOverflow=off  InputSameDT=off
  Out : Outport
  wires:
  Lokalne/1 -> Wybor/3
  [XV307SP] -> Wybor/1
  [TrybSter] -> Wybor/2
  Wybor/1 -> GUIMon/1
  GUIMon/1 -> Out/1

== system BrowarModel/Kadz filtracji/XV312 ==
  note: Sterowanie
  GUIMon : Gain
  Lokalne : Constant
  Wybor : Switch  Threshold=0.5  SaturateOnIntegerOverflow=off  InputSameDT=off
  Out : Outport
  wires:
  GUIMon/1 -> Out/1
  Wybor/1 -> GUIMon/1
  [TrybSter] -> Wybor/2
  [XV312] -> Wybor/1
  Lokalne/1 -> Wybor/3

== system BrowarModel/Kadz warzelna/ET404 ==
  note: Przetwornik pomiarowy
  In : Inport
  F_gain : Gain  Gain=0
  F_offset : Constant  Value=0
  GUIMon : Gain
  Kompensacja : Constant  Value=Kompensacja
  Product : Product  RndMeth=Zero
  Saturation : Saturate  UpperLimit=100  LowerLimit=0
  Skalowanie (0-100%) : Gain  Gain=100/SrcZakres
  Sum{,1..3} (4 alike) : Sum  Inputs=|++
  Transfer Fcn : TransferFcn  Denominator=[0.3 1]
  Zaklocenia pomiarowe : Subsystem
  Zakres : Constant  Value=Zakres/100
  Out : Outport
  wires:
  Transfer Fcn/1 -> Saturation/1
  F_offset/1 -> Sum3/2
  F_gain/1 -> Sum2/2
  Product/1 -> Sum/1
  Zakres/1 -> Product/2
  Kompensacja/1 -> Sum/2
  Sum/1 -> GUIMon/1
  Skalowanie (0-100%)/1 -> Sum1/1
  Zaklocenia pomiarowe/1(Out) -> Sum1/2
  Sum1/1 -> F_gain/1, Sum2/1
  Sum3/1 -> Transfer Fcn/1
  Sum2/1 -> Sum3/1
  In/1 -> Skalowanie (0-100%)/1
  GUIMon/1 -> Out/1
  Saturation/1 -> Product/1

== system BrowarModel/Kadz warzelna/FV404 ==
  note: Sterowanie
  GUIMon : Gain
  Lokalne : Constant  Value=0
  Wybor : Switch  Threshold=0.5  SaturateOnIntegerOverflow=off  InputSameDT=off
  Out : Outport
  wires:
  GUIMon/1 -> Out/1
  Wybor/1 -> GUIMon/1
  [TrybSter] -> Wybor/2
  [FV404] -> Wybor/1
  Lokalne/1 -> Wybor/3

== system BrowarModel/Kadz warzelna/FV404SP ==
  note: Sterowanie
  GUIMon : Gain
  Lokalne : Constant  Value=100
  Wybor : Switch  Threshold=0.5  SaturateOnIntegerOverflow=off  InputSameDT=off
  Out : Outport
  wires:
  Lokalne/1 -> Wybor/3
  [FV404SP] -> Wybor/1
  [TrybSter] -> Wybor/2
  Wybor/1 -> GUIMon/1
  GUIMon/1 -> Out/1

== system BrowarModel/Kadz warzelna/FV405 ==
  note: Sterowanie
  GUIMon : Gain
  Lokalne : Constant  Value=0
  Wybor : Switch  Threshold=0.5  SaturateOnIntegerOverflow=off  InputSameDT=off
  Out : Outport
  wires:
  Lokalne/1 -> Wybor/3
  [FV405] -> Wybor/1
  [TrybSter] -> Wybor/2
  Wybor/1 -> GUIMon/1
  GUIMon/1 -> Out/1

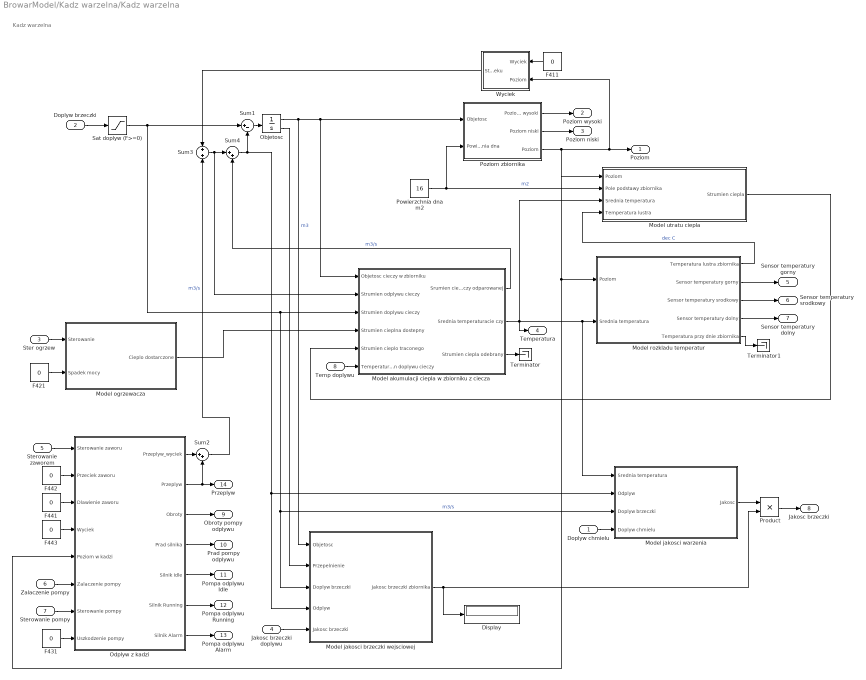
== system BrowarModel/Kadz warzelna/Kadz warzelna ==
  note: Kadz warzelna
  Doplyw chmielu : Inport
  Doplyw brzeczki : Inport  Port=2
  Ster ogrzew : Inport  Port=3
  Jakosc brzeczki doplywu : Inport  Port=4
  Sterowanie zaworem : Inport  Port=5
  Zalaczenie pompy : Inport  Port=6
  Sterowanie pompy : Inport  Port=7
  Temp doplywu : Inport  Port=8
  Display : Display
  F{411,421,431,441..443} (6 alike) : Constant  Value=0
  Model akumulacji ciepla w zbiorniku z ciecza : Subsystem
  Model jakosci brzeczki wejsciowej : Subsystem
  Model jakosci warzenia : Subsystem
  Model ogrzewacza : Subsystem
  Model rozkladu temperatur : Subsystem
  Model utratu ciepla : Subsystem
  Objetosc : Integrator  InitialCondition=0.001  LimitOutput=on  UpperSaturationLimit=48  LowerSaturationLimit=0.001  ShowSaturationPort=on
  Odplyw z kadzi : Subsystem
  Powierzchnia dna m2 : Constant  Value=16
  Poziom zbiornika : Subsystem
  Product : Product  RndMeth=Zero
  Sat doplyw (F>=0) : Saturate  UpperLimit=inf  LowerLimit=0
  Sum1 : Sum  Inputs=|+-
  Sum2 : Sum  Inputs=|++
  Sum3 : Sum
  Sum4 : Sum  Inputs=|++
  Terminator : Terminator
  Terminator1 : Terminator
  Wyciek : Subsystem
  Poziom : Outport
  Poziom wysoki : Outport  Port=2
  Poziom niski : Outport  Port=3
  Temperatura : Outport  Port=4
  Sensor temperatury gorny : Outport  Port=5
  Sensor temperatury srodkowy : Outport  Port=6
  Sensor temperatury dolny : Outport  Port=7
  Jakosc brzeczki : Outport  Port=8
  Obroty pompy odplywu : Outport  Port=9
  Prad pompy odplywu : Outport  Port=10
  Pompa odplywu Idle : Outport  Port=11
  Pompa odplywu Running : Outport  Port=12
  Pompa odplywu Alarm : Outport  Port=13
  Przeplyw : Outport  Port=14
  wires:
  Model rozkladu temperatur/4(Sensor temperatury dolny) -> Sensor temperatury dolny/1
  Model rozkladu temperatur/3(Sensor temperatury srodkowy) -> Sensor temperatury srodkowy/1
  Model rozkladu temperatur/2(Sensor temperatury gorny) -> Sensor temperatury gorny/1
  Model rozkladu temperatur/1(Temperatura lustra zbiornika) -> Model utratu ciepla/4(Temperatura lustra)  "dec C"
  Model utratu ciepla/1(Strumien ciepla) -> Model akumulacji ciepla w zbiorniku z ciecza/5(Strumien cieplo traconego)
  Sat doplyw (F>=0)/1 -> Sum1/1, Model akumulacji ciepla w zbiorniku z ciecza/3(Strumien doplywu cieczy), Model jakosci brzeczki wejsciowej/3(Doplyw brzeczki), Model jakosci warzenia/3(Doplyw brzeczki)  "m3/s"
  Model akumulacji ciepla w zbiorniku z ciecza/2(Srednia temperaturacie czy) -> Model utratu ciepla/3(Srednia temperatura), Model rozkladu temperatur/2(Srednia temperatura), Model jakosci warzenia/1(Srednia temperatura), Temperatura/1
  Powierzchnia dna m2/1 -> Model utratu ciepla/2(Pole podstawy zbiornika), Poziom zbiornika/2(Powierzchnia dna)  "m2"
  Poziom zbiornika/2(Poziom niski) -> Poziom niski/1
  Poziom zbiornika/1(Poziom  wysoki) -> Poziom wysoki/1
  Doplyw brzeczki/1 -> Sat doplyw (F>=0)/1
  Objetosc/1 -> Model akumulacji ciepla w zbiorniku z ciecza/1(Objetosc cieczy w zbiorniku), Poziom zbiornika/1(Objetosc), Model jakosci brzeczki wejsciowej/1(Objetosc)  "m3"
  Poziom zbiornika/3(Poziom) -> Model utratu ciepla/1(Poziom), Poziom/1, Wyciek/2(Poziom), Model rozkladu temperatur/1(Poziom), Odplyw z kadzi/5(Poziom w kadzi)
  Model akumulacji ciepla w zbiorniku z ciecza/1(Srumien cieczy odparowanej) -> Sum4/2  "m3/s"
  Temp doplywu/1 -> Model akumulacji ciepla w zbiorniku z ciecza/6(Temperatura strumien doplywu cieczy)
  Ster ogrzew/1 -> Model ogrzewacza/1(Sterowanie)
  F411/1 -> Wyciek/1(Wyciek)
  Sum2/1 -> Sum3/2  "m3/s"
  Sum3/1 -> Model akumulacji ciepla w zbiorniku z ciecza/2(Strumien odplywu cieczy), Sum4/1
  Wyciek/1(Strumien wycieku) -> Sum3/1
  Objetosc/2 -> Model jakosci brzeczki wejsciowej/2(Przepelnienie)
  Jakosc brzeczki doplywu/1 -> Model jakosci brzeczki wejsciowej/5(Jakosc brzeczki)
  Sum1/1 -> Objetosc/1
  Sum4/1 -> Sum1/2, Model jakosci brzeczki wejsciowej/4(Odplyw), Model jakosci warzenia/2(Odplyw)
  Doplyw chmielu/1 -> Model jakosci warzenia/4(Doplyw chmielu)
  Model jakosci warzenia/1(Jakosc) -> Product/1
  Product/1 -> Jakosc brzeczki/1
  Model jakosci brzeczki wejsciowej/1(Jakosc brzeczki zbiornika) -> Product/2, Display/1
  Model ogrzewacza/1(Cieplo dostarczone) -> Model akumulacji ciepla w zbiorniku z ciecza/4(Strumien cieplna dostepny)
  F421/1 -> Model ogrzewacza/2(Spadek mocy)
  Model akumulacji ciepla w zbiorniku z ciecza/3(Strumien ciepla odebrany) -> Terminator/1
  Model rozkladu temperatur/5(Temperatura przy dnie zbiornika) -> Terminator1/1
  F442/1 -> Odplyw z kadzi/2(Przeciek zaworu)
  F441/1 -> Odplyw z kadzi/3(Dlawienie zaworu)
  F431/1 -> Odplyw z kadzi/8(Uszkodzenie pompy)
  Sterowanie zaworem/1 -> Odplyw z kadzi/1(Sterowanie zaworu)
  Zalaczenie pompy/1 -> Odplyw z kadzi/6(Zalaczenie pompy)
  Sterowanie pompy/1 -> Odplyw z kadzi/7(Sterowanie pompy)
  F443/1 -> Odplyw z kadzi/4(Wyciek)
  Odplyw z kadzi/4(Prad silnika) -> Prad pompy odplywu/1
  Odplyw z kadzi/5(Silnik Idle) -> Pompa odplywu Idle/1
  Odplyw z kadzi/6(Silnik Running) -> Pompa odplywu Running/1
  Odplyw z kadzi/7(Silnik Alarm) -> Pompa odplywu Alarm/1
  Odplyw z kadzi/3(Obroty) -> Obroty pompy odplywu/1
  Odplyw z kadzi/2(Przeplyw) -> Sum2/2, Przeplyw/1
  Odplyw z kadzi/1(Przeplyw_wyciek) -> Sum2/1

== system BrowarModel/Kadz warzelna/LT401 ==
  note: Przetwornik pomiarowy
  In : Inport
  F_gain : Gain  Gain=0
  F_offset : Constant  Value=0
  GUIMon : Gain
  Kompensacja : Constant  Value=Kompensacja
  Product : Product  RndMeth=Zero
  Saturation : Saturate  UpperLimit=100  LowerLimit=0
  Skalowanie (0-100%) : Gain  Gain=100/SrcZakres
  Sum{,1..3} (4 alike) : Sum  Inputs=|++
  Transfer Fcn : TransferFcn  Denominator=[0.3 1]
  Zaklocenia pomiarowe : Subsystem
  Zakres : Constant  Value=Zakres/100
  Out : Outport
  wires:
  Saturation/1 -> Product/1
  GUIMon/1 -> Out/1
  In/1 -> Skalowanie (0-100%)/1
  Sum2/1 -> Sum3/1
  Sum3/1 -> Transfer Fcn/1
  Sum1/1 -> Sum2/1, F_gain/1
  Zaklocenia pomiarowe/1(Out) -> Sum1/2
  Skalowanie (0-100%)/1 -> Sum1/1
  Sum/1 -> GUIMon/1
  Kompensacja/1 -> Sum/2
  Zakres/1 -> Product/2
  Product/1 -> Sum/1
  F_gain/1 -> Sum2/2
  F_offset/1 -> Sum3/2
  Transfer Fcn/1 -> Saturation/1

== system BrowarModel/Kadz warzelna/LT401H ==
  note: Przetwornik pomiarowy
  In : Inport
  FT : Constant  Value=0
  FT_value : Constant  Value=0
  GUIMon : Gain
  Switch : Switch  Threshold=0.5  SaturateOnIntegerOverflow=off  InputSameDT=off
  Out : Outport
  wires:
  In/1 -> Switch/3
  GUIMon/1 -> Out/1
  FT/1 -> Switch/2
  Switch/1 -> GUIMon/1
  FT_value/1 -> Switch/1

== system BrowarModel/Kadz warzelna/LT401L ==
  note: Przetwornik pomiarowy
  In : Inport
  FT : Constant  Value=0
  FT_value : Constant  Value=0
  GUIMon : Gain
  Switch : Switch  Threshold=0.5  SaturateOnIntegerOverflow=off  InputSameDT=off
  Out : Outport
  wires:
  FT_value/1 -> Switch/1
  Switch/1 -> GUIMon/1
  FT/1 -> Switch/2
  GUIMon/1 -> Out/1
  In/1 -> Switch/3

== system BrowarModel/Kadz warzelna/ST404 ==
  note: Przetwornik pomiarowy
  In : Inport
  F_gain : Gain  Gain=0
  F_offset : Constant  Value=0
  GUIMon : Gain
  Kompensacja : Constant  Value=Kompensacja
  Product : Product  RndMeth=Zero
  Saturation : Saturate  UpperLimit=100  LowerLimit=0
  Skalowanie (0-100%) : Gain  Gain=100/SrcZakres
  Sum{,1..3} (4 alike) : Sum  Inputs=|++
  Transfer Fcn : TransferFcn  Denominator=[0.3 1]
  Zaklocenia pomiarowe : Subsystem
  Zakres : Constant  Value=Zakres/100
  Out : Outport
  wires:
  Saturation/1 -> Product/1
  GUIMon/1 -> Out/1
  In/1 -> Skalowanie (0-100%)/1
  Sum2/1 -> Sum3/1
  Sum3/1 -> Transfer Fcn/1
  Sum1/1 -> Sum2/1, F_gain/1
  Zaklocenia pomiarowe/1(Out) -> Sum1/2
  Skalowanie (0-100%)/1 -> Sum1/1
  Sum/1 -> GUIMon/1
  Kompensacja/1 -> Sum/2
  Zakres/1 -> Product/2
  Product/1 -> Sum/1
  F_gain/1 -> Sum2/2
  F_offset/1 -> Sum3/2
  Transfer Fcn/1 -> Saturation/1

== system BrowarModel/Kadz warzelna/TT402H ==
  note: Przetwornik pomiarowy
  In : Inport
  F_gain : Gain  Gain=0
  F_offset : Constant  Value=0
  GUIMon : Gain
  Kompensacja : Constant  Value=Kompensacja
  Product : Product  RndMeth=Zero
  Saturation : Saturate  UpperLimit=100  LowerLimit=0
  Skalowanie (0-100%) : Gain  Gain=100/SrcZakres
  Sum{,1..3} (4 alike) : Sum  Inputs=|++
  Transfer Fcn : TransferFcn  Denominator=[0.3 1]
  Zaklocenia pomiarowe : Subsystem
  Zakres : Constant  Value=Zakres/100
  Out : Outport
  wires:
  Transfer Fcn/1 -> Saturation/1
  F_offset/1 -> Sum3/2
  F_gain/1 -> Sum2/2
  Product/1 -> Sum/1
  Zakres/1 -> Product/2
  Kompensacja/1 -> Sum/2
  Sum/1 -> GUIMon/1
  Skalowanie (0-100%)/1 -> Sum1/1
  Zaklocenia pomiarowe/1(Out) -> Sum1/2
  Sum1/1 -> F_gain/1, Sum2/1
  Sum3/1 -> Transfer Fcn/1
  Sum2/1 -> Sum3/1
  In/1 -> Skalowanie (0-100%)/1
  GUIMon/1 -> Out/1
  Saturation/1 -> Product/1

== system BrowarModel/Kadz warzelna/TT402L ==
  note: Przetwornik pomiarowy
  In : Inport
  F_gain : Gain  Gain=0
  F_offset : Constant  Value=0
  GUIMon : Gain
  Kompensacja : Constant  Value=Kompensacja
  Product : Product  RndMeth=Zero
  Saturation : Saturate  UpperLimit=100  LowerLimit=0
  Skalowanie (0-100%) : Gain  Gain=100/SrcZakres
  Sum{,1..3} (4 alike) : Sum  Inputs=|++
  Transfer Fcn : TransferFcn  Denominator=[0.3 1]
  Zaklocenia pomiarowe : Subsystem
  Zakres : Constant  Value=Zakres/100
  Out : Outport
  wires:
  Transfer Fcn/1 -> Saturation/1
  F_offset/1 -> Sum3/2
  F_gain/1 -> Sum2/2
  Product/1 -> Sum/1
  Zakres/1 -> Product/2
  Kompensacja/1 -> Sum/2
  Sum/1 -> GUIMon/1
  Skalowanie (0-100%)/1 -> Sum1/1
  Zaklocenia pomiarowe/1(Out) -> Sum1/2
  Sum1/1 -> F_gain/1, Sum2/1
  Sum3/1 -> Transfer Fcn/1
  Sum2/1 -> Sum3/1
  In/1 -> Skalowanie (0-100%)/1
  GUIMon/1 -> Out/1
  Saturation/1 -> Product/1

== system BrowarModel/Kadz warzelna/TT402M ==
  note: Przetwornik pomiarowy
  In : Inport
  F_gain : Gain  Gain=0
  F_offset : Constant  Value=0
  GUIMon : Gain
  Kompensacja : Constant  Value=Kompensacja
  Product : Product  RndMeth=Zero
  Saturation : Saturate  UpperLimit=100  LowerLimit=0
  Skalowanie (0-100%) : Gain  Gain=100/SrcZakres
  Sum{,1..3} (4 alike) : Sum  Inputs=|++
  Transfer Fcn : TransferFcn  Denominator=[0.3 1]
  Zaklocenia pomiarowe : Subsystem
  Zakres : Constant  Value=Zakres/100
  Out : Outport
  wires:
  Saturation/1 -> Product/1
  GUIMon/1 -> Out/1
  In/1 -> Skalowanie (0-100%)/1
  Sum2/1 -> Sum3/1
  Sum3/1 -> Transfer Fcn/1
  Sum1/1 -> Sum2/1, F_gain/1
  Zaklocenia pomiarowe/1(Out) -> Sum1/2
  Skalowanie (0-100%)/1 -> Sum1/1
  Sum/1 -> GUIMon/1
  Kompensacja/1 -> Sum/2
  Zakres/1 -> Product/2
  Product/1 -> Sum/1
  F_gain/1 -> Sum2/2
  F_offset/1 -> Sum3/2
  Transfer Fcn/1 -> Saturation/1

== system BrowarModel/Kadz warzelna/TV402 ==
  note: Sterowanie
  GUIMon : Gain
  Lokalne : Constant  Value=100
  Wybor : Switch  Threshold=0.5  SaturateOnIntegerOverflow=off  InputSameDT=off
  Out : Outport
  wires:
  GUIMon/1 -> Out/1
  Wybor/1 -> GUIMon/1
  [TrybSter] -> Wybor/2
  [TV402] -> Wybor/1
  Lokalne/1 -> Wybor/3

== system BrowarModel/Kadz zacierna/ET205 ==
  note: Przetwornik pomiarowy
  In : Inport
  F_gain : Gain  Gain=0
  F_offset : Constant  Value=0
  GUIMon : Gain
  Kompensacja : Constant  Value=Kompensacja
  Product : Product  RndMeth=Zero
  Saturation : Saturate  UpperLimit=100  LowerLimit=0
  Skalowanie (0-100%) : Gain  Gain=100/SrcZakres
  Sum{,1..3} (4 alike) : Sum  Inputs=|++
  Transfer Fcn : TransferFcn  Denominator=[0.3 1]
  Zaklocenia pomiarowe : Subsystem
  Zakres : Constant  Value=Zakres/100
  Out : Outport
  wires:
  Transfer Fcn/1 -> Saturation/1
  F_offset/1 -> Sum3/2
  F_gain/1 -> Sum2/2
  Product/1 -> Sum/1
  Zakres/1 -> Product/2
  Kompensacja/1 -> Sum/2
  Sum/1 -> GUIMon/1
  Skalowanie (0-100%)/1 -> Sum1/1
  Zaklocenia pomiarowe/1(Out) -> Sum1/2
  Sum1/1 -> F_gain/1, Sum2/1
  Sum3/1 -> Transfer Fcn/1
  Sum2/1 -> Sum3/1
  In/1 -> Skalowanie (0-100%)/1
  GUIMon/1 -> Out/1
  Saturation/1 -> Product/1
